simulink model "prova_FaultModel"  (R2023b)
settings: Solver=VariableStepAuto  StartTime=0.0  StopTime=50.0  RelTol=1e-3
settings Model: Creator=megan  LastModifiedBy=megan
settings DebuggingCC: InheritedTsInSrcMsg=none

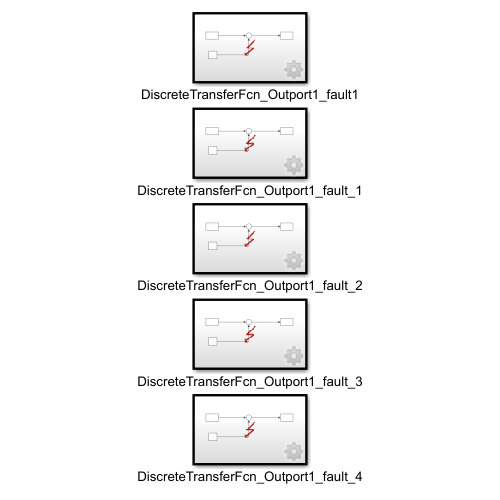
[thumbnail: Simulink's stored preview of the top-level diagram]
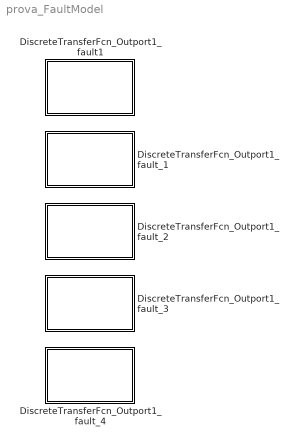
== system prova_FaultModel ==
  DiscreteTransferFcn_Outport1_fault1 : Subsystem  TreatAsAtomicUnit=on  IsInjectorSS=on
      settings: LibrarySourceBlock=mwfaultlib/Add Noise
  DiscreteTransferFcn_Outport1_fault_1 : Subsystem  TreatAsAtomicUnit=on  IsInjectorSS=on
      settings: LibrarySourceBlock=mwfaultlib/Add Noise
  DiscreteTransferFcn_Outport1_fault_2 : Subsystem  TreatAsAtomicUnit=on  IsInjectorSS=on
      settings: LibrarySourceBlock=mwfaultlib/Add Noise
  DiscreteTransferFcn_Outport1_fault_3 : Subsystem  TreatAsAtomicUnit=on  IsInjectorSS=on
      settings: LibrarySourceBlock=mwfaultlib/Add Noise
  DiscreteTransferFcn_Outport1_fault_4 : Subsystem  TreatAsAtomicUnit=on  IsInjectorSS=on
      settings: LibrarySourceBlock=mwfaultlib/Add Noise

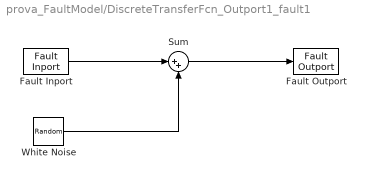
== system prova_FaultModel/DiscreteTransferFcn_Outport1_fault1 ==
  Fault Inport : FaultInport
  Fault Outport : FaultOutport
  Sum : Sum  Inputs=|++  OutDataTypeStr=Inherit: Inherit via back propagation
  White Noise : RandomNumber  DisableCoverage=on  Variance=0.01  Seed=[23341]
  wires:
  White Noise/1 -> Sum/2
  Sum/1 -> Fault Outport/1
  Fault Inport/1 -> Sum/1

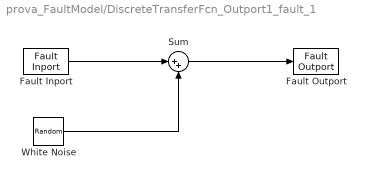
== system prova_FaultModel/DiscreteTransferFcn_Outport1_fault_1 ==
  Fault Inport : FaultInport
  Fault Outport : FaultOutport
  Sum : Sum  Inputs=|++  OutDataTypeStr=Inherit: Inherit via back propagation
  White Noise : RandomNumber  DisableCoverage=on  Variance=0.1  Seed=[23341]
  wires:
  White Noise/1 -> Sum/2
  Sum/1 -> Fault Outport/1
  Fault Inport/1 -> Sum/1

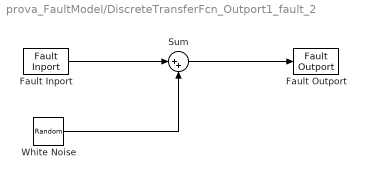
== system prova_FaultModel/DiscreteTransferFcn_Outport1_fault_2 ==
  Fault Inport : FaultInport
  Fault Outport : FaultOutport
  Sum : Sum  Inputs=|++  OutDataTypeStr=Inherit: Inherit via back propagation
  White Noise : RandomNumber  DisableCoverage=on  Seed=[23341]
  wires:
  White Noise/1 -> Sum/2
  Sum/1 -> Fault Outport/1
  Fault Inport/1 -> Sum/1

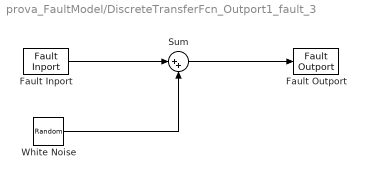
== system prova_FaultModel/DiscreteTransferFcn_Outport1_fault_3 ==
  Fault Inport : FaultInport
  Fault Outport : FaultOutport
  Sum : Sum  Inputs=|++  OutDataTypeStr=Inherit: Inherit via back propagation
  White Noise : RandomNumber  DisableCoverage=on  Variance=10  Seed=[23341]
  wires:
  White Noise/1 -> Sum/2
  Sum/1 -> Fault Outport/1
  Fault Inport/1 -> Sum/1

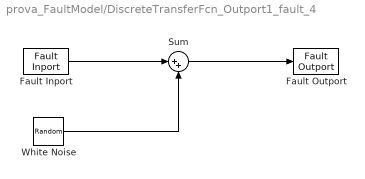
== system prova_FaultModel/DiscreteTransferFcn_Outport1_fault_4 ==
  Fault Inport : FaultInport
  Fault Outport : FaultOutport
  Sum : Sum  Inputs=|++  OutDataTypeStr=Inherit: Inherit via back propagation
  White Noise : RandomNumber  DisableCoverage=on  Variance=100  Seed=[23341]
  wires:
  White Noise/1 -> Sum/2
  Sum/1 -> Fault Outport/1
  Fault Inport/1 -> Sum/1
